simulink model "TrayectoriaPurePursuitM"  (R2023b)
settings: Solver=FixedStepDiscrete  StartTime=0.0  StopTime=51  FixedStep=0.01  MaxStep=0.01  RelTol=1e-3  EnableMultiTasking=on
model workspace (MAT data in the model file):
  d = 0.223
libraries: slpidlib x1
settings Model: ExtModeTrigDuration=2  Creator=Manuel  LastModifiedBy=Manuel
settings OptimizationCC: EnhancedBackFolding=on  PassReuseOutputArgsAs=Individual arguments  ZeroExternalMemoryAtStartup=off  ZeroInternalMemoryAtStartup=off  MaxStackSize=64  OptimizeBlockOrder=speed  DifferentSizesBufferReuse=on  EfficientTunableParamExpr=on
settings DebuggingCC: ParameterTunabilityLossMsg=error
settings HardwareCC: ProdBitPerInt=16  ProdBitPerPointer=16  ProdBitPerSizeT=16  ProdBitPerPtrDiffT=16  ProdLargestAtomicFloat=None  ProdWordSize=8  ProdHWDeviceType=Atmel->AVR
settings SFSimCC: MATLABDynamicMemAlloc=off
settings RTWCC: Description=Embedded Coder  SystemTargetFile=ert.tlc  HardwareBoard=Arduino Mega 2560  TemplateMakefile=ert_default_tmf  Toolchain=Arduino AVR  BuildConfiguration=Faster Runs
settings CodeAppCC: ForceParamTrailComments=on  IgnoreCustomStorageClasses=off  OperatorAnnotations=on  SimulinkDataObjDesc=on  SFDataObjDesc=on  InsertBlockDesc=on
settings ERTTargetCC: SupportContinuousTime=on  SupportVariableSizeSignals=on  ExtModeTransport=3  ExtModeStaticAlloc=on  ExtModeAutomaticAllocSize=off  ExtModeStaticAllocSize=2048  ExtModeMexFile=ext_xcp  ExtModeIntrfLevel=Level2 - Open

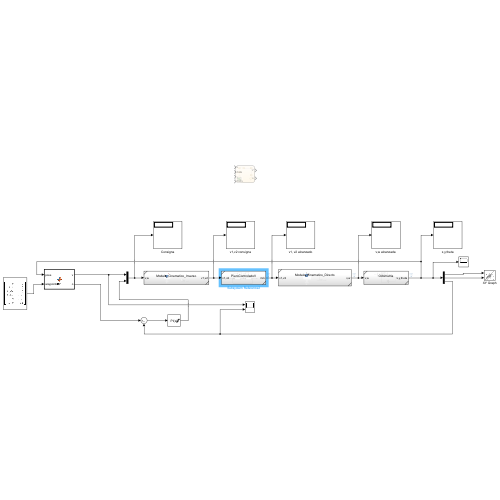
[thumbnail: Simulink's stored preview of the top-level diagram]
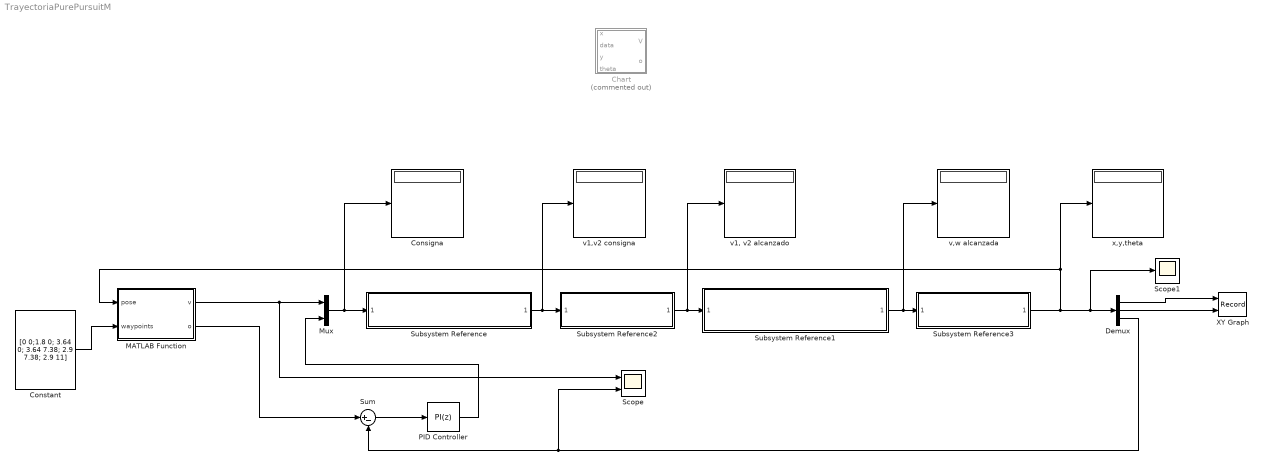
== system TrayectoriaPurePursuitM ==
  Chart : Stateflow chart  Commented=on  TreatAsAtomicUnit=on
  Consigna : Display
  Constant : Constant  Value=[0 0;1.8 0; 3.64 0; 3.64 7.38; 2.9 7.38; 2.9 11]
  Demux : Demux  Outputs=3
  MATLAB Function : MATLAB Function  TreatAsAtomicUnit=on
  Mux : Mux  Inputs=2
  PID Controller : slpidlib/PID Controller  Controller=PI  Form=Parallel  TimeDomain=Discrete-time  UseExternalTs=off  SampleTime=-1  IntegratorMethod=Forward Euler  FilterMethod=Forward Euler  ControllerParametersSource=internal  P=28.7152388371894  I=11.8097265226966  UseKiTs=off  D=0.183724426277108  N=2.90189397027696  UseFilter=on  TunerSelectOption=Transfer Function Based (PID Tuner App)  InitialConditionSource=internal  InitialConditionForIntegrator=0  InitialConditionForFilter=0  DifferentiatorICPrevScaledInput=0  ExternalReset=none  TrackingMode=off  Kt=1  LimitOutput=on  SatLimitsSource=internal  UpperSaturationLimit=pi  LowerSaturationLimit=-pi  LinearizeAsGain=on  AntiWindupMode=back-calculation  Kb=0.9  LimitIntegrator=off  UpperIntegratorSaturationLimit=inf  LowerIntegratorSaturationLimit=-inf  POutMin=[]  POutMax=[]  IOutMin=[]  IOutMax=[]  DOutMin=[]  DOutMax=[]  NOutMin=[]  NOutMax=[]  SumOutMin=[]  SumOutMax=[]  SaturationOutMin=[]  SaturationOutMax=[]  PParamMin=[]  PParamMax=[]  IParamMin=[]  IParamMax=[]  DParamMin=[]  DParamMax=[]  NParamMin=[]  NParamMax=[]  KbParamMin=[]  KbParamMax=[]  KtParamMin=[]  KtParamMax=[]  KbOutMin=[]  KbOutMax=[]  KtOutMin=[]  KtOutMax=[]  IntegratorOutMin=[]  IntegratorOutMax=[]  FilterOutMin=[]  FilterOutMax=[]  SumI1OutMin=[]  SumI1OutMax=[]  SumI2OutMin=[]  SumI2OutMax=[]  SumI3OutMin=[]  SumI3OutMax=[]  SumI4OutMin=[]  SumI4OutMax=[]  SumDOutMin=[]  SumDOutMax=[]  DifferentiatorOutMin=[]  DifferentiatorOutMax=[]  FilterDiffOutCoefMin=[]  FilterDiffOutCoefMax=[]  ReciprocalOutMin=[]  ReciprocalOutMax=[]  SumDenOutMin=[]  SumDenOutMax=[]  SumNumOutMin=[]  SumNumOutMax=[]  DivideOutMin=[]  DivideOutMax=[]  UdiffTsProdOutMin=[]  UdiffTsProdOutMax=[]  NTsProdOutMin=[]  NTsProdOutMax=[]  UintegralTsProdOutMin=[]  UintegralTsProdOutMax=[]  UngainTsProdOutMin=[]  UngainTsProdOutMax=[]  ClampingZeroOutDataTypeStr=Inherit: Inherit via back propagation  ClampingZeroOutMin=[]  ClampingZeroOutMax=[]  FilterDenConstantOutDataTypeStr=Inherit: Inherit via back propagation  FilterDenConstantOutMin=[]  FilterDenConstantOutMax=[]  PCopyOutDataTypeStr=Inherit: Inherit via back propagation  PCopyOutMin=[]  PCopyOutMax=[]  NCopyOutDataTypeStr=Inherit: Inherit via back propagation  NCopyOutMin=[]  NCopyOutMax=[]  IntegratorContinuousStateAttributes=''  IntegratorStateMustResolveToSignalObject=off  IntegratorRTWStateStorageClass=Auto  FilterContinuousStateAttributes=''  FilterStateMustResolveToSignalObject=off  FilterRTWStateStorageClass=Auto  ParallelPVariant=InternalParameters  IdealPVariant=Disabled  IVariant=InternalParameters  DVariant=Disabled  IntegratorVariant=Discrete  SatVariant=Enabled  AWVariant=BackCalculation  PCopyVariant=Disabled  TRVariant=Disabled  FdbkBlocksVariant=Forward  IdealPFdbkVariant=Disabled  SatFdbkVariant=Disabled  DerivativeFilterVariant=Disabled  NVariant=Disabled  NCopyVariant=Disabled_SignalSpec  FilterICVariant=Disabled  IntegratorICVariant=InternalICs  ExternalResetVariant=Disabled  TRSumVariant=Passthrough  SumFdbkVariant=Disabled  SumVariant=Sum_PI  TsampFilterVariant=InternalTs  TsampNgainVariant=Passthrough  TsampIntegralVariant=Disabled_SignalSpec  ExternalSaturationOutDataTypeStr=Inherit: Same as second input
  Scope : Scope  NumInputPorts=2
  Scope1 : Scope
  Subsystem Reference : Subsystem  ReferencedSubsystem=Modelo_Cinematico_Inverso
  Subsystem Reference1 : Subsystem  ReferencedSubsystem=Modelo_Cinematico_Directo
  Subsystem Reference2 : Subsystem  ReferencedSubsystem=PieroControladoV
  Subsystem Reference3 : Subsystem  ReferencedSubsystem=Odometria
  Sum : Sum  Inputs=|+-
  XY Graph : Record  FileSettingsInternal="{\"entries\":[{\"content\":{\"excelSettings\":{\"content\":{},\"type\":\"Streamout.ExcelSettings\"}},\"type\":\"Streamout.FileSettingStorage\",\"uuid\":\"\"}],\"packageUris\":[\"http:\\/\\/schema.mathworks.com\\/mf0\\/streamout_blocks\\/R2020a\"],\"version\":\"1.0\"}"  Layout=[1 1]  SignalsInternal="{\"entries\":[{\"content\":{\"signals\":[{\"content\":{\"blockPath\":[],\"dimensions\":[1],\"domain\":\"\",\"lineColor\":\"#a2142f\",\"plots\":[1],\"port\":1,\"sid\":[\"36\"],\"signalID\":1433,\"signalName\":\"Demux:1\"},\"type\":\"RecordBlkView.Signal\",\"uuid\":\"\"},{\"content\":{\"blockPath\":[],\"dimensions\":[1],\"domain\":\"\",\"lineColor\":\"#139fff\",\"plots\":[1],\"port\":2,\"sid\":[\"36\"],\"signalID\":1437,\"signalName\":\"Demux:2\"},\"type\":\"RecordBlkView.Signal\",\"uuid\":\"\"}]},\"type\":\"RecordBlkView.InputSignals\",\"uuid\":\"\"}],\"packageUris\":[\"http:\\/\\/schema.mathworks.com\\/mf0\\/streamout_blocks\\/R2020a\"],\"version\":\"1.0\"}"  VisualizationBindings="{\"xyplotplugin\":{\"info\":[{\"series\":[{\"bindingParametersList\":[{\"parameter\":\"X-Axis\",\"signalID\":1433,\"signalName\":\"Demux:1\"},{\"parameter\":\"Y-Axis\",\"signalID\":1437,\"signalName\":\"Demux:2\"}],\"seriesID\":3305}],\"subplotID\":1}]}}"  CompatibilityTag=XY
  "v,w alcanzada " : Display
  "v1, v2 alcanzado" : Display
  v1,v2 consigna : Display
  x,y,theta : Display
  wires:
  Subsystem Reference1/1 -> "v,w alcanzada "/1, Subsystem Reference3/1
  Subsystem Reference/1 -> v1,v2 consigna/1, Subsystem Reference2/1
  Subsystem Reference2/1 -> "v1, v2 alcanzado"/1, Subsystem Reference1/1
  Subsystem Reference3/1 -> MATLAB Function/1(pose), x,y,theta/1, Scope1/1, Demux/1
  Demux/1 -> XY Graph/1
  Demux/2 -> XY Graph/2
  Demux/3 -> Scope/2, Sum/2
  Mux/1 -> Consigna/1, Subsystem Reference/1
  Sum/1 -> PID Controller/1
  PID Controller/1 -> Mux/2
  MATLAB Function/2(o) -> Sum/1
  Constant/1 -> MATLAB Function/2(waypoints)
  MATLAB Function/1(v) -> Scope/1, Mux/1

== matlab function TrayectoriaPurePursuitM/MATLAB Function ==
  data: v output; pose input; o output; waypoints input
function [v, o] = fcn(pose, waypoints)

    LookAhead=0.22;
    persistent indice;

    if isempty(indice)
        indice=1;
    end

    v=0.3;
    x=pose(1);
    y=pose(2);
    tamano=length(waypoints);
    if(tamano >= indice)
        distancia=sqrt((waypoints(indice,1)-x)^2+(waypoints(indice,2)-y)^2);
        while ((distancia < LookAhead) && (tamano>indice))
            indice=indice+1;
            distancia=sqrt((waypoints(indice,1)-x)^2+(waypoints(indice,2)-y)^2);
            v=0.1;
        end
        o=atan2(waypoints(indice,2)-y,waypoints(indice,1)-x);
    else
        o=pose(3);
        v=0;
    end
    indice;
    
end

== stateflow chart TrayectoriaPurePursuitM/Chart ==
  state GiroIzquierda2
    entry:
    V=0.08;
    o=-pi;
  state Marcha2
    entry:
    V=0.3;
    o=-pi/2;
  state GiroIzquierda1
    entry:
    V=0.08;
    o=-pi/2;
  state Marcha3
    entry:
    V=0.3;
    o=-pi;
  state Marcha1
    entry:
    V=0.3;
    o=0;
  state Fin
    entry:
    V=0;
    o=-pi;
  state Inicio
    entry:
    V=0;
    o=0;
  Marcha2 -> GiroIzquierda2 : [y<-1.2]
  GiroIzquierda1 -> Marcha2 : [theta<-pi/2]
  GiroIzquierda2 -> Marcha3 : [theta<-pi]
  Marcha1 -> GiroIzquierda1 : [x>2.1]
  Marcha3 -> Fin : [x<1]
  Inicio -> Marcha1 : after(1,sec)
  (default) -> Inicio
  data: V output double size=1; o output double size=1; x input double size=1; data input; y input double size=1; theta input double size=1
